simulink model "PD_400MHz"  (R2017b)
settings: Solver=FixedStepDiscrete  StartTime=0.0  StopTime=1e-3  FixedStep=1/Fs  RelTol=1e-3
values from neighbouring files (symbols this model uses):
  Fs = 100    [main.m]    (also in plot_alias.m = 1000; plot_fft.m = 1000; plot_fft_filter.m = 1000; plot_filtering.m = 10000)
libraries: Library_SignalGeneration x10
settings Model: Creator=Keith  LastModifiedBy=Keith

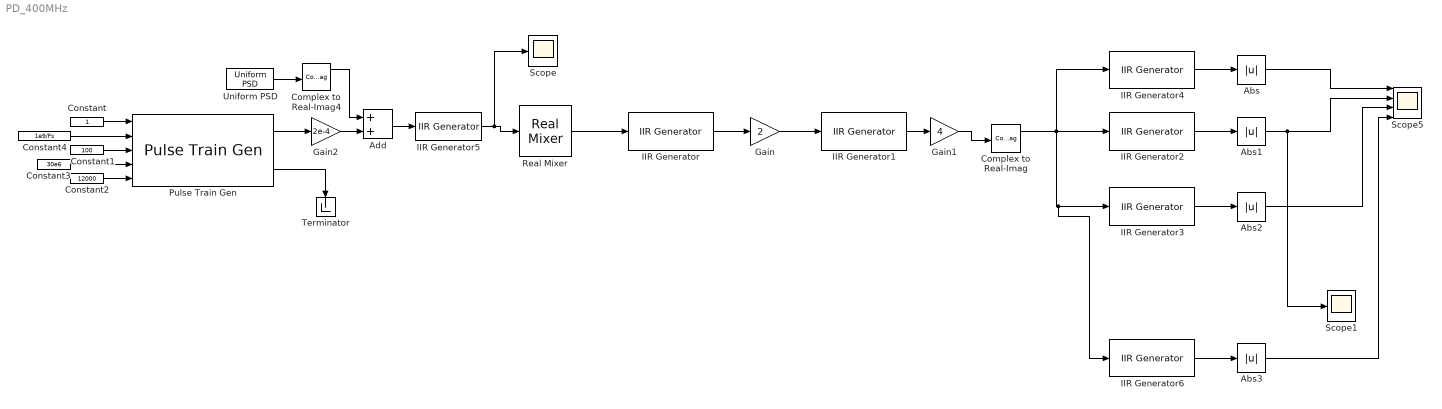
== system PD_400MHz ==
  Abs{,1..3} (4 alike) : Abs
  Add : Sum
  Complex to Real-Imag : ComplexToRealImag
  Complex to Real-Imag4 : ComplexToRealImag
  Constant : Constant
  Constant1 : Constant  Value=100
  Constant2 : Constant  Value=12000
  Constant3 : Constant  Value=30e6
  Constant4 : Constant  Value=1e9/Fs
  Gain : Gain  Gain=2
  Gain1 : Gain  Gain=4
  Gain2 : Gain  Gain=2e-4
  IIR Generator : Library_SignalGeneration/IIR Generator  ihFilename=Mix_LPF_6 Pole Inv Cheby LPF.txt  shiftEnable=off  shiftFactor=0.5  bodeplt=0
      settings: AttributesFormatString=|
      | IIR File:  %<ihFilename>
      | Quad Shift: %<shiftEnable>,%<shiftFactor>
  IIR Generator1 : Library_SignalGeneration/IIR Generator  ihFilename=PRF_BandPass.txt  shiftEnable=on  shiftFactor=(2e6)/Fs  bodeplt=0
      settings: AttributesFormatString=|
      | IIR File:  %<ihFilename>
      | Quad Shift: %<shiftEnable>,%<shiftFactor>
  IIR Generator2 : Library_SignalGeneration/IIR Generator  ihFilename=DOP_BandPass.txt  shiftEnable=on  shiftFactor=2e6/Fs  bodeplt=0
      settings: AttributesFormatString=|
      | IIR File:  %<ihFilename>
      | Quad Shift: %<shiftEnable>,%<shiftFactor>
  IIR Generator3 : Library_SignalGeneration/IIR Generator  ihFilename=DOP_BandPass.txt  shiftEnable=on  shiftFactor=(2e6+1200)/Fs  bodeplt=0
      settings: AttributesFormatString=|
      | IIR File:  %<ihFilename>
      | Quad Shift: %<shiftEnable>,%<shiftFactor>
  IIR Generator4 : Library_SignalGeneration/IIR Generator  ihFilename=DOP_BandPass.txt  shiftEnable=on  shiftFactor=(2e6-1200)/Fs  bodeplt=0
      settings: AttributesFormatString=|
      | IIR File:  %<ihFilename>
      | Quad Shift: %<shiftEnable>,%<shiftFactor>
  IIR Generator5 : Library_SignalGeneration/IIR Generator  ihFilename=FE_BandPass.txt  shiftEnable=off  shiftFactor=0.5  bodeplt=0
      settings: AttributesFormatString=|
      | IIR File:  %<ihFilename>
      | Quad Shift: %<shiftEnable>,%<shiftFactor>
  IIR Generator6 : Library_SignalGeneration/IIR Generator  ihFilename=DOP_BandPass.txt  shiftEnable=on  shiftFactor=(2e6+4000)/Fs  bodeplt=0
      settings: AttributesFormatString=|
      | IIR File:  %<ihFilename>
      | Quad Shift: %<shiftEnable>,%<shiftFactor>
  Pulse Train Gen : Library_SignalGeneration/Pulse Train Gen
  Real Mixer : Library_SignalGeneration/Real Mixer  loFrequencyHz=28e6+12000
      settings: AttributesFormatString=LO: %<loFrequencyHz>
  Scope : Scope
  Scope1 : Scope
  Scope5 : Scope  NumInputPorts=4
  Terminator : Terminator
  Uniform PSD : Library_SignalGeneration/Uniform PSD  nzdb=4.5  reftemp=290  Fs=Fs
  wires:
  Pulse Train Gen/2 -> Terminator/1
  Constant/1 -> Pulse Train Gen/1
  Constant1/1 -> Pulse Train Gen/3
  Constant3/1 -> Pulse Train Gen/4
  Constant4/1 -> Pulse Train Gen/2
  Real Mixer/1 -> IIR Generator/1
  IIR Generator/1 -> Gain/1
  Constant2/1 -> Pulse Train Gen/5
  IIR Generator1/1 -> Gain1/1
  Gain/1 -> IIR Generator1/1
  Gain1/1 -> Complex to Real-Imag/1
  Complex to Real-Imag/1 -> IIR Generator6/1, IIR Generator3/1, IIR Generator4/1, IIR Generator2/1
  Pulse Train Gen/1 -> Gain2/1
  Gain2/1 -> Add/2
  Uniform PSD/1 -> Complex to Real-Imag4/1
  Complex to Real-Imag4/1 -> Add/1
  Add/1 -> IIR Generator5/1
  IIR Generator5/1 -> Scope/1, Real Mixer/1
  IIR Generator4/1 -> Abs/1
  IIR Generator3/1 -> Abs2/1
  IIR Generator2/1 -> Abs1/1
  IIR Generator6/1 -> Abs3/1
  Abs/1 -> Scope5/1
  Abs1/1 -> Scope1/1, Scope5/2
  Abs2/1 -> Scope5/3
  Abs3/1 -> Scope5/4
